simulink model "Disturbance_models_fixed"  (R2022a)
settings: Solver=ode45  StartTime=0.0  StopTime=50  RelTol=1e-3
values from neighbouring files (symbols this model uses):
  A = [0 0 1 0 0 ... (first row only)    [DesignProjectP2.m]    (also in DesignProjectP3.m; DesignProject_OffsetP3.m; mpc_example_regulation.m = [ 	 0,       0,              1,  0, 0; 	 0,       0,        ; mpc_example_tracking.m = [ 	 0,       0,              1,  0, 0; 	 0,       0,        )
  absolute_encoder_counts_per_revolution = 128    [ELEN90064_Project_Parameters.m]
  B = [0;0;0;0;1/La]    [DesignProjectP2.m]    (also in DesignProjectP3.m; DesignProject_OffsetP3.m; mpc_example_regulation.m = [0; 0; 0; 0; 1/La]; mpc_example_tracking.m = [0; 0; 0; 0; 1/La])
  C = [1 0 0 0 0 ... (first row only)    [DesignProjectP2.m]    (also in DesignProjectP3.m; DesignProject_OffsetP3.m; mpc_example_regulation.m; mpc_example_tracking.m)
  init = [theta_m_init; theta_l_init; thetadot_m_init; thetadot_l_init; Ia_init]    [ELEN90064_Project_Parameters.m]
  K_sin = K_dist(1:5)    [DesignProjectP2.m]    (also in DesignProject_OffsetP3.m = K_dist(7:8))
  Kd_sin = K_dist(6:7)    [DesignProjectP2.m]
  L = place(A', C', observer_poles)'    [DesignProjectP2.m]    (also in DesignProjectP3.m; DesignProject_OffsetP3.m = L_t'; phase2_emc.m = place(A',C',desired_obsv_poles)')
  theta_l_init = deg2rad(0)    [ELEN90064_Project_Parameters.m]    (also in mpc_example_regulation.m; mpc_example_tracking.m)
  vision_fps = 50    [ELEN90064_Project_Parameters.m]
  w = 2*pi*1/4    (= 1.57079632679)    [DesignProjectP2.m]    (also in DesignProject_OffsetP3.m)
settings Model: Creator=Admin  LastModifiedBy=Admin

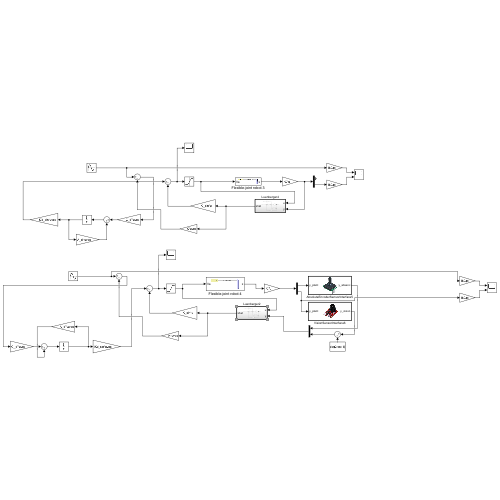
[thumbnail: Simulink's stored preview of the top-level diagram]
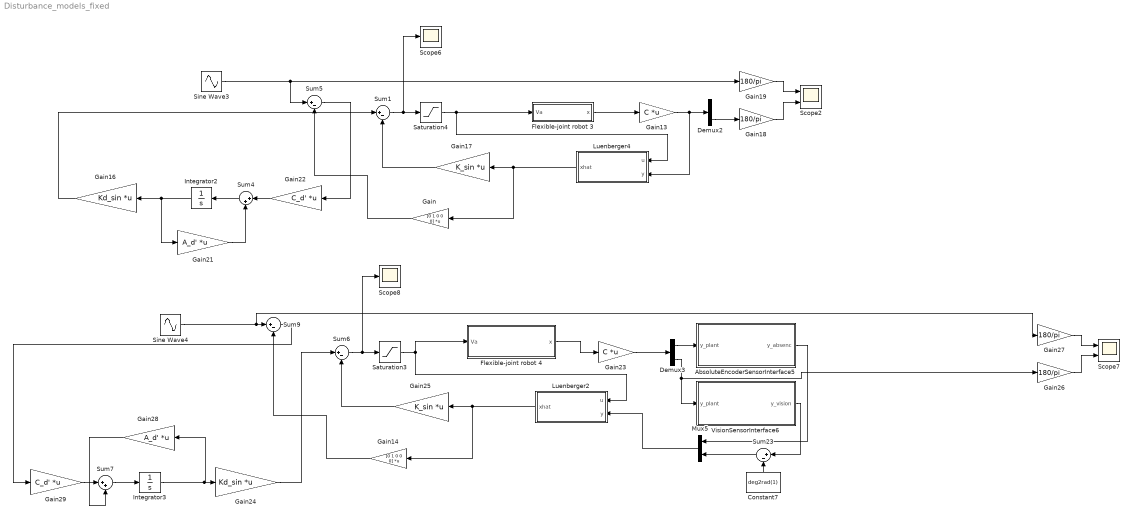
== system Disturbance_models_fixed ==
  AbsoluteEncoderSensorInterface5 : Subsystem  TreatAsAtomicUnit=on
      mask Display: image('$imagefile'); % Use "Edit Image" on toolstrip to change.
  Constant7 : Constant  Value=deg2rad(1)
  Demux2 : Demux  Outputs=2
  Demux3 : Demux  Outputs=2
  Flexible-joint robot 3 : Subsystem
      mask Display: image('$imagefile'); % Use "Edit Image" on toolstrip to change.
  Flexible-joint robot 4 : Subsystem
      mask Display: image('$imagefile'); % Use "Edit Image" on toolstrip to change.
  Gain : Gain  Gain=[0 1 0 0 0]  Multiplication=Matrix(K*u) (u vector)
  Gain13 : Gain  Gain=C  Multiplication=Matrix(K*u)
  Gain14 : Gain  Gain=[0 1 0 0 0]  Multiplication=Matrix(K*u) (u vector)
  Gain16 : Gain  Gain=Kd_sin  Multiplication=Matrix(K*u) (u vector)
  Gain17 : Gain  Gain=K_sin  Multiplication=Matrix(K*u)
  Gain{18..19,26..27} (4 alike) : Gain  Gain=180/pi
  Gain21 : Gain  Gain=A_d'  Multiplication=Matrix(K*u) (u vector)
  Gain22 : Gain  Gain=C_d'  Multiplication=Matrix(K*u) (u vector)
  Gain23 : Gain  Gain=C  Multiplication=Matrix(K*u)
  Gain24 : Gain  Gain=Kd_sin  Multiplication=Matrix(K*u) (u vector)
  Gain25 : Gain  Gain=K_sin  Multiplication=Matrix(K*u)
  Gain28 : Gain  Gain=A_d'  Multiplication=Matrix(K*u) (u vector)
  Gain29 : Gain  Gain=C_d'  Multiplication=Matrix(K*u) (u vector)
  Integrator2 : Integrator
  Integrator3 : Integrator
  Luenberger2 : Subsystem  TreatAsAtomicUnit=on
  Luenberger4 : Subsystem  TreatAsAtomicUnit=on
  Mux5 : Mux  Inputs=2
  Saturation3 : Saturate  UpperLimit=6  LowerLimit=-6
  Saturation4 : Saturate  UpperLimit=6  LowerLimit=-6
  Scope2 : Scope  NumInputPorts=2
  Scope6 : Scope
  Scope7 : Scope  NumInputPorts=2
  Scope8 : Scope
  Sine Wave3 : Sin  Amplitude=deg2rad(30)  Frequency=w  Phase=deg2rad(30)  SampleTime=0
  Sine Wave4 : Sin  Amplitude=deg2rad(30)  Frequency=w  Phase=deg2rad(30)  SampleTime=0
  Sum{1,5..6,9,23} (5 alike) : Sum  Inputs=|+-
  Sum4 : Sum  Inputs=|++
  Sum7 : Sum  Inputs=|++
  VisionSensorInterface6 : Subsystem  TreatAsAtomicUnit=on
      mask Display: image('$imagefile'); % Use "Edit Image" on toolstrip to change.
  wires:
  Sine Wave3/1 -> Sum5/1, Gain19/1
  Gain19/1 -> Scope2/1
  Flexible-joint robot 3/1(x) -> Gain13/1
  Gain18/1 -> Scope2/2
  Gain17/1 -> Sum1/2
  Luenberger4/1(xhat) -> Gain/1, Gain17/1
  Gain13/1 -> Luenberger4/2(y), Demux2/1
  Demux2/2 -> Gain18/1
  Sum4/1 -> Integrator2/1
  Gain22/1 -> Sum4/1
  Sum1/1 -> Saturation4/1, Scope6/1
  Gain21/1 -> Sum4/2
  Gain16/1 -> Sum1/1
  Integrator2/1 -> Gain16/1, Gain21/1
  Gain/1 -> Sum5/2
  Sum5/1 -> Gain22/1
  Sum23/1 -> Mux5/2
  AbsoluteEncoderSensorInterface5/1(y_absenc) -> Mux5/1
  VisionSensorInterface6/1(y_vision) -> Sum23/1
  Demux3/1 -> AbsoluteEncoderSensorInterface5/1(y_plant)
  Constant7/1 -> Sum23/2
  Sum9/1 -> Gain29/1
  Gain14/1 -> Sum9/2
  Integrator3/1 -> Gain28/1, Gain24/1
  Gain24/1 -> Sum6/1
  Gain28/1 -> Sum7/2
  Sum6/1 -> Scope8/1, Saturation3/1
  Gain29/1 -> Sum7/1
  Sum7/1 -> Integrator3/1
  Demux3/2 -> Gain26/1, VisionSensorInterface6/1(y_plant)
  Gain23/1 -> Demux3/1
  Luenberger2/1(xhat) -> Gain25/1, Gain14/1
  Gain25/1 -> Sum6/2
  Gain26/1 -> Scope7/2
  Flexible-joint robot 4/1(x) -> Gain23/1
  Gain27/1 -> Scope7/1
  Sine Wave4/1 -> Gain27/1, Sum9/1
  Mux5/1 -> Luenberger2/2(y)
  Saturation3/1 -> Flexible-joint robot 4/1(Va), Luenberger2/1(u)
  Saturation4/1 -> Luenberger4/1(u), Flexible-joint robot 3/1(Va)

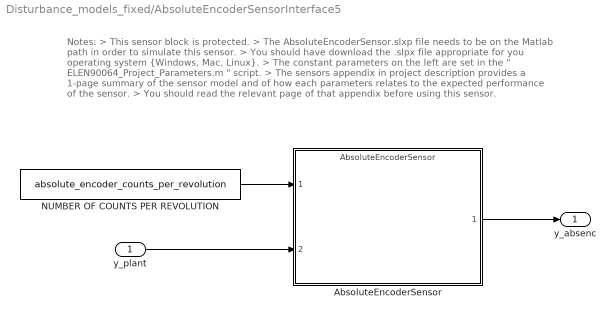
== system Disturbance_models_fixed/AbsoluteEncoderSensorInterface5 ==
  note: Notes:
      | > This sensor block is protected.
      | > The AbsoluteEncoderSensor.slxp file needs to be on the Matlab path in order to simulate this sensor.
      | > You should have download the .slpx file appropriate for you operating system {Windows, Mac, Linux}.
      | > The constant parameters on the left are set in the " ELEN90064_Project_Parameters.m " script.
      | > The sensors appendix in project description provides a 1-page summary of the sensor model and of how each parameters relates to the expected performance of the sensor.
      | > You should read the relevant page of that appendix before using this sensor.
  y_plant : Inport
  AbsoluteEncoderSensor : ModelReference  ModelNameDialog=AbsoluteEncoderSensor.slxp  ModelReferenceVersion=1.16  CopyOfModelProtected=on
  NUMBER OF COUNTS PER REVOLUTION : Constant  Value=absolute_encoder_counts_per_revolution
  y_absenc : Outport
  wires:
  NUMBER OF COUNTS PER REVOLUTION/1 -> AbsoluteEncoderSensor/1
  y_plant/1 -> AbsoluteEncoderSensor/2
  AbsoluteEncoderSensor/1 -> y_absenc/1

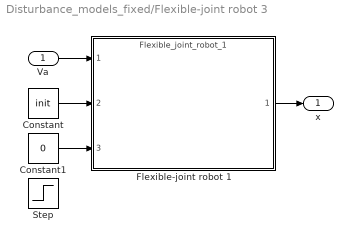
== system Disturbance_models_fixed/Flexible-joint robot 3 ==
  Va : Inport
  Constant : Constant  Value=init
  Constant1 : Constant  Value=0
  Flexible-joint robot 1 : ModelReference  ModelNameDialog=Flexible_joint_robot_1  ModelReferenceVersion=1.65  CopyOfModelProtected=on
  Step : Step  After=0.05  SampleTime=0
  x : Outport
  wires:
  Constant/1 -> Flexible-joint robot 1/2
  Flexible-joint robot 1/1 -> x/1
  Va/1 -> Flexible-joint robot 1/1
  Constant1/1 -> Flexible-joint robot 1/3

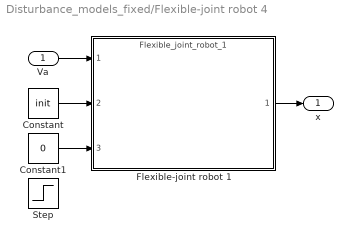
== system Disturbance_models_fixed/Flexible-joint robot 4 ==
  Va : Inport
  Constant : Constant  Value=init
  Constant1 : Constant  Value=0
  Flexible-joint robot 1 : ModelReference  ModelNameDialog=Flexible_joint_robot_1  ModelReferenceVersion=1.65  CopyOfModelProtected=on
  Step : Step  After=0.05  SampleTime=0
  x : Outport
  wires:
  Constant1/1 -> Flexible-joint robot 1/3
  Va/1 -> Flexible-joint robot 1/1
  Flexible-joint robot 1/1 -> x/1
  Constant/1 -> Flexible-joint robot 1/2

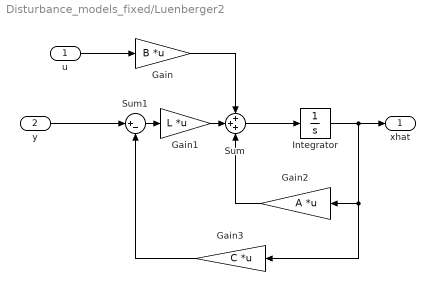
== system Disturbance_models_fixed/Luenberger2 ==
  u : Inport
  y : Inport  Port=2
  Gain : Gain  Gain=B  Multiplication=Matrix(K*u) (u vector)
  Gain1 : Gain  Gain=L  Multiplication=Matrix(K*u) (u vector)
  Gain2 : Gain  Gain=A  Multiplication=Matrix(K*u) (u vector)
  Gain3 : Gain  Gain=C  Multiplication=Matrix(K*u) (u vector)
  Integrator : Integrator
  Sum : Sum  Inputs=+++
  Sum1 : Sum  Inputs=|+-
  xhat : Outport
  wires:
  Gain3/1 -> Sum1/2
  Gain2/1 -> Sum/3
  Integrator/1 -> xhat/1, Gain2/1, Gain3/1
  Sum/1 -> Integrator/1
  Gain1/1 -> Sum/2
  Sum1/1 -> Gain1/1
  y/1 -> Sum1/1
  Gain/1 -> Sum/1
  u/1 -> Gain/1

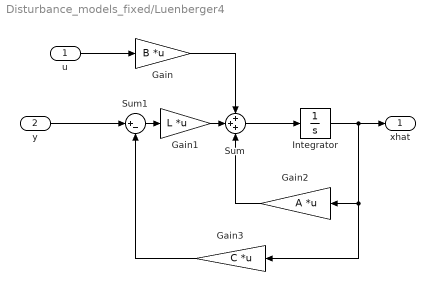
== system Disturbance_models_fixed/Luenberger4 ==
  u : Inport
  y : Inport  Port=2
  Gain : Gain  Gain=B  Multiplication=Matrix(K*u) (u vector)
  Gain1 : Gain  Gain=L  Multiplication=Matrix(K*u) (u vector)
  Gain2 : Gain  Gain=A  Multiplication=Matrix(K*u) (u vector)
  Gain3 : Gain  Gain=C  Multiplication=Matrix(K*u) (u vector)
  Integrator : Integrator
  Sum : Sum  Inputs=+++
  Sum1 : Sum  Inputs=|+-
  xhat : Outport
  wires:
  u/1 -> Gain/1
  Gain/1 -> Sum/1
  y/1 -> Sum1/1
  Sum1/1 -> Gain1/1
  Gain1/1 -> Sum/2
  Sum/1 -> Integrator/1
  Integrator/1 -> Gain3/1, Gain2/1, xhat/1
  Gain2/1 -> Sum/3
  Gain3/1 -> Sum1/2

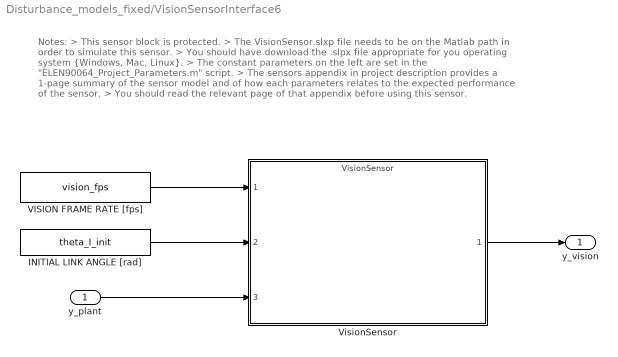
== system Disturbance_models_fixed/VisionSensorInterface6 ==
  note: Notes:
      | > This sensor block is protected.
      | > The VisionSensor.slxp file needs to be on the Matlab path in order to simulate this sensor.
      | > You should have download the .slpx file appropriate for you operating system {Windows, Mac, Linux}.
      | > The constant parameters on the left are set in the "ELEN90064_Project_Parameters.m" script.
      | > The sensors appendix in project description provides a 1-page summary of the sensor model and of how each parameters relates to the expected performance of the sensor.
      | > You should read the relevant page of that appendix before using this sensor.
  y_plant : Inport
  INITIAL LINK ANGLE [rad] : Constant  Value=theta_l_init
  VISION FRAME RATE [fps] : Constant  Value=vision_fps
  VisionSensor : ModelReference  ModelNameDialog=VisionSensor.slxp  ModelReferenceVersion=1.19  CopyOfModelProtected=on
  y_vision : Outport
  wires:
  VisionSensor/1 -> y_vision/1
  y_plant/1 -> VisionSensor/3
  INITIAL LINK ANGLE [rad]/1 -> VisionSensor/2
  VISION FRAME RATE [fps]/1 -> VisionSensor/1
